simulink model "model_NW_feedback_EXCITATORY_INPUT_INCREASE_FIRING"  (R2020b)
settings: Solver=VariableStepAuto  StartTime=0.0  StopTime=20.0  RelTol=1e-3
libraries: simulink x1
settings Model: Creator=Isabel  LastModifiedBy=Isabel

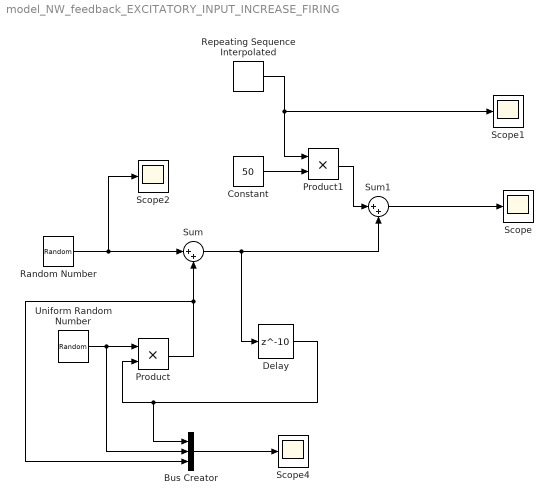
== system model_NW_feedback_EXCITATORY_INPUT_INCREASE_FIRING ==
  Bus Creator : BusCreator  Inputs=3
  Constant : Constant  Value=50
  Delay : Delay  DelayLength=10  InitialCondition=0
  Product : Product
  Product1 : Product
  Random Number : RandomNumber  Mean=3  SampleTime=0.05
  Repeating Sequence Interpolated : simulink/Sources/Repeating Sequence Interpolated  OutValues=[0 0 0 0.025 0.075 0.1 0.2 0.3 0.5 0.615 0.7 0.68 0.6 0.2 0.1 0.05 0.02 0 0 0 0].'  TimeValues=[0 0.1 0.2 0.25 0.3 0.35 0.425 0.475 0.55 0.6 0.65 0.68 0.71 0.78 0.81 0.85 0.9 1 1.1 1.2 5].'  LookUpMeth=Interpolation-Use End Values  tsamp=0.005  OutMin=[]  OutMax=[]  OutDataTypeStr=double  OutputDataTypeScalingMode=double  OutDataType=fixdt(0,8)  OutScaling=2^-10
  Scope{,1..2,4} (4 alike) : Scope
  Sum : Sum  Inputs=|++
  Sum1 : Sum  Inputs=|++
  Uniform Random Number : UniformRandomNumber  Minimum=0  SampleTime=0.1
  wires:
  Uniform Random Number/1 -> Bus Creator/2, Product/1
  Random Number/1 -> Scope2/1, Sum/1
  Product/1 -> Sum/2, Bus Creator/3
  Repeating Sequence Interpolated/1 -> Scope1/1, Product1/1
  Sum/1 -> Delay/1, Sum1/2
  Sum1/1 -> Scope/1
  Bus Creator/1 -> Scope4/1
  Delay/1 -> Bus Creator/1, Product/2
  Product1/1 -> Sum1/1
  Constant/1 -> Product1/2
